simulink model "TST_EngBrk_ECRCtl"  (R2016b)
settings: Solver=FixedStepDiscrete  StartTime=0.0  StopTime=simTime  FixedStep=sampleTime  RelTol=1e-3
values from neighbouring files (symbols this model uses):
  testCase = 1    [initTST_EngBrk_ECRCtl_001.m]    (also in initTST_EngBrk_ECRCtl_002.m = 2; initTST_EngBrk_ECRCtl_003.m = 3; initTST_EngBrk_ECRCtl_004.m = 4)
libraries: simulink x5
settings Model: Creator=WF305  LastModifiedBy=WF305
settings DebuggingCC: SignalRangeChecking=error

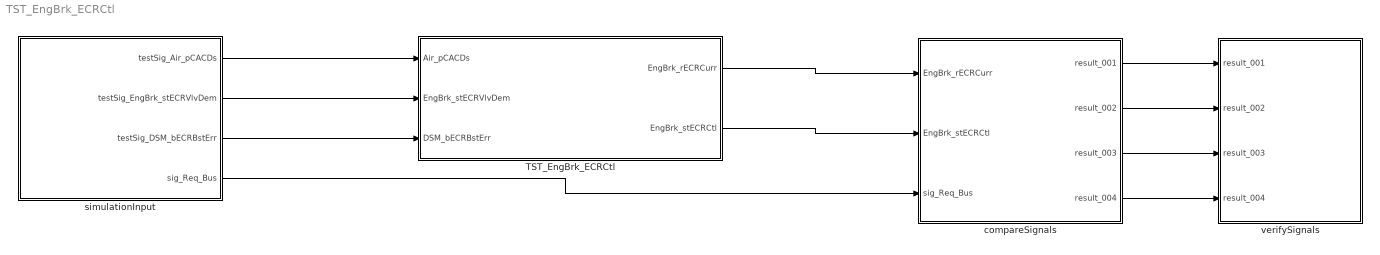
== system TST_EngBrk_ECRCtl ==
  TST_EngBrk_ECRCtl : Subsystem
  compareSignals : Subsystem
  simulationInput : Subsystem
  verifySignals : Subsystem
  wires:
  simulationInput/1(testSig_Air_pCACDs) -> TST_EngBrk_ECRCtl/1(Air_pCACDs)
  simulationInput/2(testSig_EngBrk_stECRVlvDem) -> TST_EngBrk_ECRCtl/2(EngBrk_stECRVlvDem)
  simulationInput/3(testSig_DSM_bECRBstErr) -> TST_EngBrk_ECRCtl/3(DSM_bECRBstErr)
  TST_EngBrk_ECRCtl/1(EngBrk_rECRCurr) -> compareSignals/1(EngBrk_rECRCurr)
  TST_EngBrk_ECRCtl/2(EngBrk_stECRCtl) -> compareSignals/2(EngBrk_stECRCtl)
  simulationInput/4(sig_Req_Bus) -> compareSignals/3(sig_Req_Bus)
  compareSignals/1(result_001) -> verifySignals/1(result_001)
  compareSignals/2(result_002) -> verifySignals/2(result_002)
  compareSignals/3(result_003) -> verifySignals/3(result_003)
  compareSignals/4(result_004) -> verifySignals/4(result_004)

== system TST_EngBrk_ECRCtl/TST_EngBrk_ECRCtl ==
  Air_pCACDs : Inport
  EngBrk_stECRVlvDem : Inport  Port=2
  DSM_bECRBstErr : Inport  Port=3
  EngBrk_ECRCtl : ModelReference  ModelNameDialog=EngBrk_ECRCtl  ModelReferenceVersion=1.8  TriggerPortName=function  TriggerPortTriggerType=function-call  TriggerPortStatesWhenEnabling=held
  Function_Call : simulink/Ports & Subsystems/Function-Call Generator  sample_time=sampleTime  numberOfIterations=1
  EngBrk_rECRCurr : Outport
  EngBrk_stECRCtl : Outport  Port=2
  wires:
  Function_Call/1 -> EngBrk_ECRCtl/Trigger
  Air_pCACDs/1 -> EngBrk_ECRCtl/1
  EngBrk_stECRVlvDem/1 -> EngBrk_ECRCtl/2
  DSM_bECRBstErr/1 -> EngBrk_ECRCtl/3
  EngBrk_ECRCtl/1 -> EngBrk_rECRCurr/1
  EngBrk_ECRCtl/2 -> EngBrk_stECRCtl/1

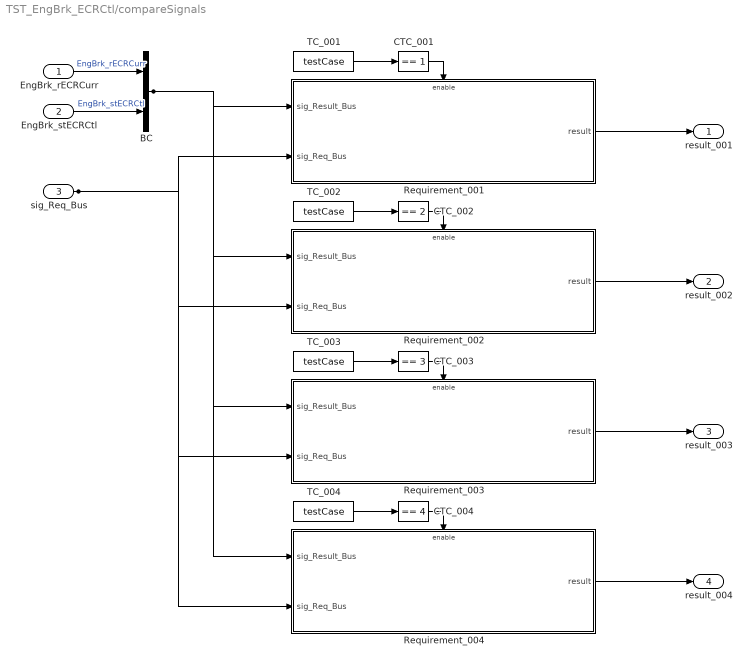
== system TST_EngBrk_ECRCtl/compareSignals ==
  EngBrk_rECRCurr : Inport
  EngBrk_stECRCtl : Inport  Port=2
  sig_Req_Bus : Inport  Port=3
  BC : BusCreator  Inputs=2
  CTC_001 : simulink/Logic and Bit Operations/Compare To Constant  relop===  const=1  OutDataTypeStr=boolean
  CTC_002 : simulink/Logic and Bit Operations/Compare To Constant  relop===  const=2  OutDataTypeStr=boolean
  CTC_003 : simulink/Logic and Bit Operations/Compare To Constant  relop===  const=3  OutDataTypeStr=boolean
  CTC_004 : simulink/Logic and Bit Operations/Compare To Constant  relop===  const=4  OutDataTypeStr=boolean
  Requirement_001 : Subsystem
  Requirement_002 : Subsystem
  Requirement_003 : Subsystem
  Requirement_004 : Subsystem
  TC_001 : Constant  Value=testCase
  TC_002 : Constant  Value=testCase
  TC_003 : Constant  Value=testCase
  TC_004 : Constant  Value=testCase
  result_001 : Outport
  result_002 : Outport  Port=2
  result_003 : Outport  Port=3
  result_004 : Outport  Port=4
  wires:
  EngBrk_rECRCurr/1 -> BC/1  "EngBrk_rECRCurr"
  EngBrk_stECRCtl/1 -> BC/2  "EngBrk_stECRCtl"
  TC_001/1 -> CTC_001/1
  CTC_001/1 -> Requirement_001/Enable
  sig_Req_Bus/1 -> Requirement_001/2(sig_Req_Bus), Requirement_002/2(sig_Req_Bus), Requirement_003/2(sig_Req_Bus), Requirement_004/2(sig_Req_Bus)
  BC/1 -> Requirement_001/1(sig_Result_Bus), Requirement_002/1(sig_Result_Bus), Requirement_003/1(sig_Result_Bus), Requirement_004/1(sig_Result_Bus)
  Requirement_001/1(result) -> result_001/1
  TC_002/1 -> CTC_002/1
  CTC_002/1 -> Requirement_002/Enable
  Requirement_002/1(result) -> result_002/1
  TC_003/1 -> CTC_003/1
  CTC_003/1 -> Requirement_003/Enable
  Requirement_003/1(result) -> result_003/1
  TC_004/1 -> CTC_004/1
  CTC_004/1 -> Requirement_004/Enable
  Requirement_004/1(result) -> result_004/1

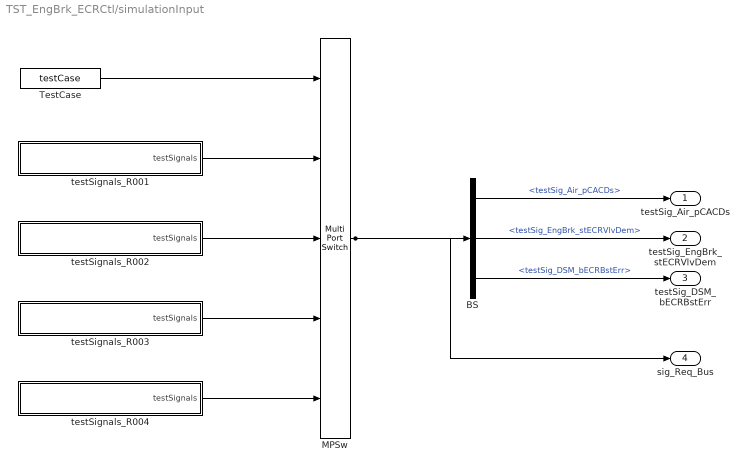
== system TST_EngBrk_ECRCtl/simulationInput ==
  BS : BusSelector  OutputSignals=testSig_Air_pCACDs,testSig_EngBrk_stECRVlvDem,testSig_DSM_bECRBstErr
  MPSw : MultiPortSwitch  Inputs=4  SaturateOnIntegerOverflow=on  InputSameDT=on
  TestCase : Constant  Value=testCase
  testSignals_R001 : Subsystem
  testSignals_R002 : Subsystem
  testSignals_R003 : Subsystem
  testSignals_R004 : Subsystem
  testSig_Air_pCACDs : Outport
  testSig_EngBrk_stECRVlvDem : Outport  Port=2
  testSig_DSM_bECRBstErr : Outport  Port=3
  sig_Req_Bus : Outport  Port=4
  wires:
  BS/1 -> testSig_Air_pCACDs/1  "<testSig_Air_pCACDs>"
  BS/2 -> testSig_EngBrk_stECRVlvDem/1  "<testSig_EngBrk_stECRVlvDem>"
  BS/3 -> testSig_DSM_bECRBstErr/1  "<testSig_DSM_bECRBstErr>"
  MPSw/1 -> BS/1, sig_Req_Bus/1
  TestCase/1 -> MPSw/1
  testSignals_R001/1(testSignals) -> MPSw/2
  testSignals_R002/1(testSignals) -> MPSw/3
  testSignals_R003/1(testSignals) -> MPSw/4
  testSignals_R004/1(testSignals) -> MPSw/5

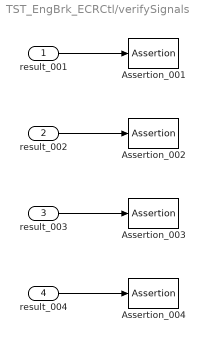
== system TST_EngBrk_ECRCtl/verifySignals ==
  result_001 : Inport
  result_002 : Inport  Port=2
  result_003 : Inport  Port=3
  result_004 : Inport  Port=4
  Assertion_001 : Assertion  Enabled=off
  Assertion_002 : Assertion  Enabled=off
  Assertion_003 : Assertion  Enabled=off
  Assertion_004 : Assertion  Enabled=off
  wires:
  result_001/1 -> Assertion_001/1
  result_002/1 -> Assertion_002/1
  result_003/1 -> Assertion_003/1
  result_004/1 -> Assertion_004/1

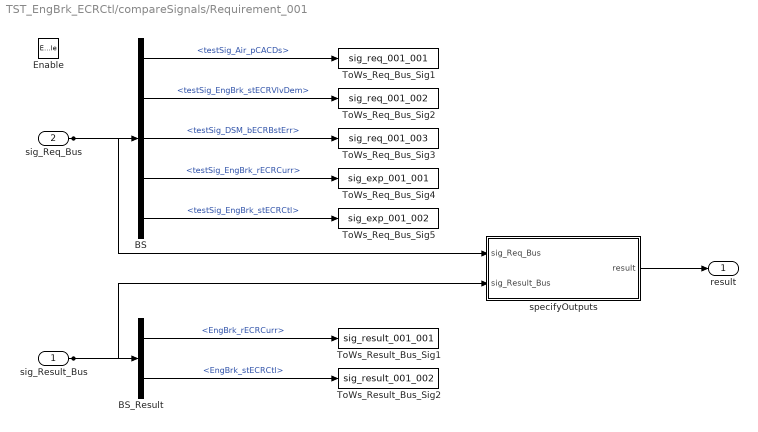
== system TST_EngBrk_ECRCtl/compareSignals/Requirement_001 ==
  sig_Result_Bus : Inport
  sig_Req_Bus : Inport  Port=2
  Enable : EnablePort
  BS : BusSelector  OutputSignals=testSig_Air_pCACDs,testSig_EngBrk_stECRVlvDem,testSig_DSM_bECRBstErr,testSig_EngBrk_rECRCurr,testSig_EngBrk_stECRCtl
  BS_Result : BusSelector  OutputSignals=EngBrk_rECRCurr,EngBrk_stECRCtl
  ToWs_Req_Bus_Sig1 : ToWorkspace  VariableName=sig_req_001_001  SaveFormat=Structure With Time
  ToWs_Req_Bus_Sig2 : ToWorkspace  VariableName=sig_req_001_002  SaveFormat=Structure With Time
  ToWs_Req_Bus_Sig3 : ToWorkspace  VariableName=sig_req_001_003  SaveFormat=Structure With Time
  ToWs_Req_Bus_Sig4 : ToWorkspace  VariableName=sig_exp_001_001  SaveFormat=Structure With Time
  ToWs_Req_Bus_Sig5 : ToWorkspace  VariableName=sig_exp_001_002  SaveFormat=Structure With Time
  ToWs_Result_Bus_Sig1 : ToWorkspace  VariableName=sig_result_001_001  SaveFormat=Structure With Time
  ToWs_Result_Bus_Sig2 : ToWorkspace  VariableName=sig_result_001_002  SaveFormat=Structure With Time
  specifyOutputs : Subsystem
  result : Outport
  wires:
  sig_Req_Bus/1 -> BS/1, specifyOutputs/1(sig_Req_Bus)
  BS/1 -> ToWs_Req_Bus_Sig1/1  "<testSig_Air_pCACDs>"
  BS/2 -> ToWs_Req_Bus_Sig2/1  "<testSig_EngBrk_stECRVlvDem>"
  BS/3 -> ToWs_Req_Bus_Sig3/1  "<testSig_DSM_bECRBstErr>"
  BS/4 -> ToWs_Req_Bus_Sig4/1  "<testSig_EngBrk_rECRCurr>"
  BS/5 -> ToWs_Req_Bus_Sig5/1  "<testSig_EngBrk_stECRCtl>"
  sig_Result_Bus/1 -> BS_Result/1, specifyOutputs/2(sig_Result_Bus)
  BS_Result/1 -> ToWs_Result_Bus_Sig1/1  "<EngBrk_rECRCurr>"
  BS_Result/2 -> ToWs_Result_Bus_Sig2/1  "<EngBrk_stECRCtl>"
  specifyOutputs/1(result) -> result/1

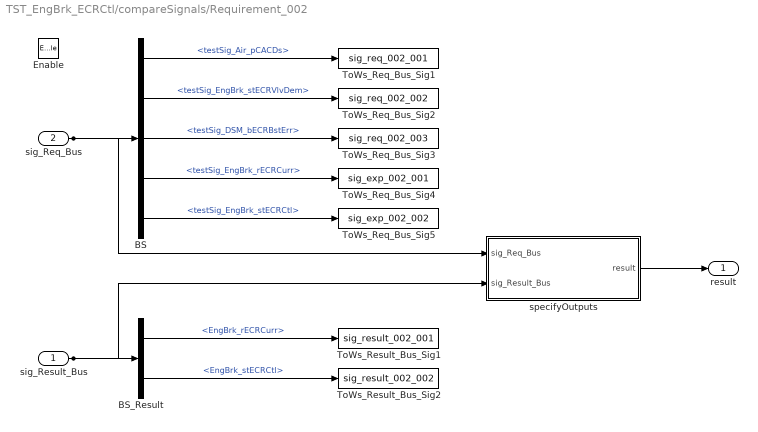
== system TST_EngBrk_ECRCtl/compareSignals/Requirement_002 ==
  sig_Result_Bus : Inport
  sig_Req_Bus : Inport  Port=2
  Enable : EnablePort
  BS : BusSelector  OutputSignals=testSig_Air_pCACDs,testSig_EngBrk_stECRVlvDem,testSig_DSM_bECRBstErr,testSig_EngBrk_rECRCurr,testSig_EngBrk_stECRCtl
  BS_Result : BusSelector  OutputSignals=EngBrk_rECRCurr,EngBrk_stECRCtl
  ToWs_Req_Bus_Sig1 : ToWorkspace  VariableName=sig_req_002_001  SaveFormat=Structure With Time
  ToWs_Req_Bus_Sig2 : ToWorkspace  VariableName=sig_req_002_002  SaveFormat=Structure With Time
  ToWs_Req_Bus_Sig3 : ToWorkspace  VariableName=sig_req_002_003  SaveFormat=Structure With Time
  ToWs_Req_Bus_Sig4 : ToWorkspace  VariableName=sig_exp_002_001  SaveFormat=Structure With Time
  ToWs_Req_Bus_Sig5 : ToWorkspace  VariableName=sig_exp_002_002  SaveFormat=Structure With Time
  ToWs_Result_Bus_Sig1 : ToWorkspace  VariableName=sig_result_002_001  SaveFormat=Structure With Time
  ToWs_Result_Bus_Sig2 : ToWorkspace  VariableName=sig_result_002_002  SaveFormat=Structure With Time
  specifyOutputs : Subsystem
  result : Outport
  wires:
  sig_Req_Bus/1 -> BS/1, specifyOutputs/1(sig_Req_Bus)
  BS/1 -> ToWs_Req_Bus_Sig1/1  "<testSig_Air_pCACDs>"
  BS/2 -> ToWs_Req_Bus_Sig2/1  "<testSig_EngBrk_stECRVlvDem>"
  BS/3 -> ToWs_Req_Bus_Sig3/1  "<testSig_DSM_bECRBstErr>"
  BS/4 -> ToWs_Req_Bus_Sig4/1  "<testSig_EngBrk_rECRCurr>"
  BS/5 -> ToWs_Req_Bus_Sig5/1  "<testSig_EngBrk_stECRCtl>"
  sig_Result_Bus/1 -> BS_Result/1, specifyOutputs/2(sig_Result_Bus)
  BS_Result/1 -> ToWs_Result_Bus_Sig1/1  "<EngBrk_rECRCurr>"
  BS_Result/2 -> ToWs_Result_Bus_Sig2/1  "<EngBrk_stECRCtl>"
  specifyOutputs/1(result) -> result/1

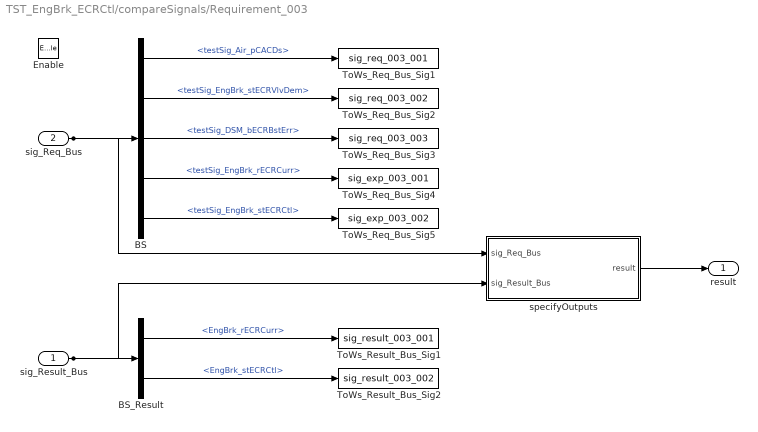
== system TST_EngBrk_ECRCtl/compareSignals/Requirement_003 ==
  sig_Result_Bus : Inport
  sig_Req_Bus : Inport  Port=2
  Enable : EnablePort
  BS : BusSelector  OutputSignals=testSig_Air_pCACDs,testSig_EngBrk_stECRVlvDem,testSig_DSM_bECRBstErr,testSig_EngBrk_rECRCurr,testSig_EngBrk_stECRCtl
  BS_Result : BusSelector  OutputSignals=EngBrk_rECRCurr,EngBrk_stECRCtl
  ToWs_Req_Bus_Sig1 : ToWorkspace  VariableName=sig_req_003_001  SaveFormat=Structure With Time
  ToWs_Req_Bus_Sig2 : ToWorkspace  VariableName=sig_req_003_002  SaveFormat=Structure With Time
  ToWs_Req_Bus_Sig3 : ToWorkspace  VariableName=sig_req_003_003  SaveFormat=Structure With Time
  ToWs_Req_Bus_Sig4 : ToWorkspace  VariableName=sig_exp_003_001  SaveFormat=Structure With Time
  ToWs_Req_Bus_Sig5 : ToWorkspace  VariableName=sig_exp_003_002  SaveFormat=Structure With Time
  ToWs_Result_Bus_Sig1 : ToWorkspace  VariableName=sig_result_003_001  SaveFormat=Structure With Time
  ToWs_Result_Bus_Sig2 : ToWorkspace  VariableName=sig_result_003_002  SaveFormat=Structure With Time
  specifyOutputs : Subsystem
  result : Outport
  wires:
  sig_Req_Bus/1 -> BS/1, specifyOutputs/1(sig_Req_Bus)
  BS/1 -> ToWs_Req_Bus_Sig1/1  "<testSig_Air_pCACDs>"
  BS/2 -> ToWs_Req_Bus_Sig2/1  "<testSig_EngBrk_stECRVlvDem>"
  BS/3 -> ToWs_Req_Bus_Sig3/1  "<testSig_DSM_bECRBstErr>"
  BS/4 -> ToWs_Req_Bus_Sig4/1  "<testSig_EngBrk_rECRCurr>"
  BS/5 -> ToWs_Req_Bus_Sig5/1  "<testSig_EngBrk_stECRCtl>"
  sig_Result_Bus/1 -> BS_Result/1, specifyOutputs/2(sig_Result_Bus)
  BS_Result/1 -> ToWs_Result_Bus_Sig1/1  "<EngBrk_rECRCurr>"
  BS_Result/2 -> ToWs_Result_Bus_Sig2/1  "<EngBrk_stECRCtl>"
  specifyOutputs/1(result) -> result/1

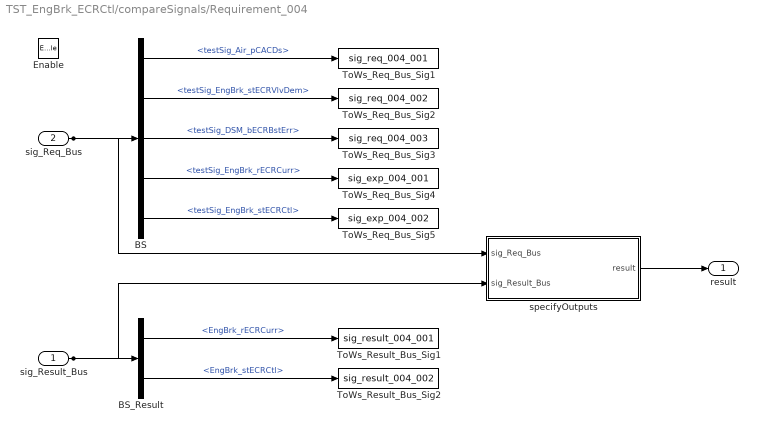
== system TST_EngBrk_ECRCtl/compareSignals/Requirement_004 ==
  sig_Result_Bus : Inport
  sig_Req_Bus : Inport  Port=2
  Enable : EnablePort
  BS : BusSelector  OutputSignals=testSig_Air_pCACDs,testSig_EngBrk_stECRVlvDem,testSig_DSM_bECRBstErr,testSig_EngBrk_rECRCurr,testSig_EngBrk_stECRCtl
  BS_Result : BusSelector  OutputSignals=EngBrk_rECRCurr,EngBrk_stECRCtl
  ToWs_Req_Bus_Sig1 : ToWorkspace  VariableName=sig_req_004_001  SaveFormat=Structure With Time
  ToWs_Req_Bus_Sig2 : ToWorkspace  VariableName=sig_req_004_002  SaveFormat=Structure With Time
  ToWs_Req_Bus_Sig3 : ToWorkspace  VariableName=sig_req_004_003  SaveFormat=Structure With Time
  ToWs_Req_Bus_Sig4 : ToWorkspace  VariableName=sig_exp_004_001  SaveFormat=Structure With Time
  ToWs_Req_Bus_Sig5 : ToWorkspace  VariableName=sig_exp_004_002  SaveFormat=Structure With Time
  ToWs_Result_Bus_Sig1 : ToWorkspace  VariableName=sig_result_004_001  SaveFormat=Structure With Time
  ToWs_Result_Bus_Sig2 : ToWorkspace  VariableName=sig_result_004_002  SaveFormat=Structure With Time
  specifyOutputs : Subsystem
  result : Outport
  wires:
  sig_Req_Bus/1 -> BS/1, specifyOutputs/1(sig_Req_Bus)
  BS/1 -> ToWs_Req_Bus_Sig1/1  "<testSig_Air_pCACDs>"
  BS/2 -> ToWs_Req_Bus_Sig2/1  "<testSig_EngBrk_stECRVlvDem>"
  BS/3 -> ToWs_Req_Bus_Sig3/1  "<testSig_DSM_bECRBstErr>"
  BS/4 -> ToWs_Req_Bus_Sig4/1  "<testSig_EngBrk_rECRCurr>"
  BS/5 -> ToWs_Req_Bus_Sig5/1  "<testSig_EngBrk_stECRCtl>"
  sig_Result_Bus/1 -> BS_Result/1, specifyOutputs/2(sig_Result_Bus)
  BS_Result/1 -> ToWs_Result_Bus_Sig1/1  "<EngBrk_rECRCurr>"
  BS_Result/2 -> ToWs_Result_Bus_Sig2/1  "<EngBrk_stECRCtl>"
  specifyOutputs/1(result) -> result/1

== system TST_EngBrk_ECRCtl/simulationInput/testSignals_R001 ==
  BC : BusCreator  Inputs=5
  spec_Air_pCACDs : FromWorkspace  VariableName=testSig_Air_pCACDs  Interpolate=off  OutputAfterFinalValue=Holding final value
  spec_DSM_bECRBstErr : FromWorkspace  VariableName=testSig_DSM_bECRBstErr  Interpolate=off  OutputAfterFinalValue=Holding final value
  spec_EngBrk_rECRCurr : FromWorkspace  VariableName=testSig_EngBrk_rECRCurr  Interpolate=off  OutputAfterFinalValue=Holding final value
  spec_EngBrk_stECRCtl : FromWorkspace  VariableName=testSig_EngBrk_stECRCtl  Interpolate=off  OutputAfterFinalValue=Holding final value
  spec_EngBrk_stECRVlvDem : FromWorkspace  VariableName=testSig_EngBrk_stECRVlvDem  Interpolate=off  OutputAfterFinalValue=Holding final value
  testSignals : Outport
  wires:
  BC/1 -> testSignals/1
  spec_Air_pCACDs/1 -> BC/1  "testSig_Air_pCACDs"
  spec_EngBrk_stECRVlvDem/1 -> BC/2  "testSig_EngBrk_stECRVlvDem"
  spec_DSM_bECRBstErr/1 -> BC/3  "testSig_DSM_bECRBstErr"
  spec_EngBrk_rECRCurr/1 -> BC/4  "testSig_EngBrk_rECRCurr"
  spec_EngBrk_stECRCtl/1 -> BC/5  "testSig_EngBrk_stECRCtl"

== system TST_EngBrk_ECRCtl/simulationInput/testSignals_R002 ==
  BC : BusCreator  Inputs=5
  spec_Air_pCACDs : FromWorkspace  VariableName=testSig_Air_pCACDs  Interpolate=off  OutputAfterFinalValue=Holding final value
  spec_DSM_bECRBstErr : FromWorkspace  VariableName=testSig_DSM_bECRBstErr  Interpolate=off  OutputAfterFinalValue=Holding final value
  spec_EngBrk_rECRCurr : FromWorkspace  VariableName=testSig_EngBrk_rECRCurr  Interpolate=off  OutputAfterFinalValue=Holding final value
  spec_EngBrk_stECRCtl : FromWorkspace  VariableName=testSig_EngBrk_stECRCtl  Interpolate=off  OutputAfterFinalValue=Holding final value
  spec_EngBrk_stECRVlvDem : FromWorkspace  VariableName=testSig_EngBrk_stECRVlvDem  Interpolate=off  OutputAfterFinalValue=Holding final value
  testSignals : Outport
  wires:
  BC/1 -> testSignals/1
  spec_Air_pCACDs/1 -> BC/1  "testSig_Air_pCACDs"
  spec_EngBrk_stECRVlvDem/1 -> BC/2  "testSig_EngBrk_stECRVlvDem"
  spec_DSM_bECRBstErr/1 -> BC/3  "testSig_DSM_bECRBstErr"
  spec_EngBrk_rECRCurr/1 -> BC/4  "testSig_EngBrk_rECRCurr"
  spec_EngBrk_stECRCtl/1 -> BC/5  "testSig_EngBrk_stECRCtl"

== system TST_EngBrk_ECRCtl/simulationInput/testSignals_R003 ==
  BC : BusCreator  Inputs=5
  spec_Air_pCACDs : FromWorkspace  VariableName=testSig_Air_pCACDs  Interpolate=off  OutputAfterFinalValue=Holding final value
  spec_DSM_bECRBstErr : FromWorkspace  VariableName=testSig_DSM_bECRBstErr  Interpolate=off  OutputAfterFinalValue=Holding final value
  spec_EngBrk_rECRCurr : FromWorkspace  VariableName=testSig_EngBrk_rECRCurr  Interpolate=off  OutputAfterFinalValue=Holding final value
  spec_EngBrk_stECRCtl : FromWorkspace  VariableName=testSig_EngBrk_stECRCtl  Interpolate=off  OutputAfterFinalValue=Holding final value
  spec_EngBrk_stECRVlvDem : FromWorkspace  VariableName=testSig_EngBrk_stECRVlvDem  Interpolate=off  OutputAfterFinalValue=Holding final value
  testSignals : Outport
  wires:
  BC/1 -> testSignals/1
  spec_Air_pCACDs/1 -> BC/1  "testSig_Air_pCACDs"
  spec_EngBrk_stECRVlvDem/1 -> BC/2  "testSig_EngBrk_stECRVlvDem"
  spec_DSM_bECRBstErr/1 -> BC/3  "testSig_DSM_bECRBstErr"
  spec_EngBrk_rECRCurr/1 -> BC/4  "testSig_EngBrk_rECRCurr"
  spec_EngBrk_stECRCtl/1 -> BC/5  "testSig_EngBrk_stECRCtl"

== system TST_EngBrk_ECRCtl/simulationInput/testSignals_R004 ==
  BC : BusCreator  Inputs=5
  spec_Air_pCACDs : FromWorkspace  VariableName=testSig_Air_pCACDs  Interpolate=off  OutputAfterFinalValue=Holding final value
  spec_DSM_bECRBstErr : FromWorkspace  VariableName=testSig_DSM_bECRBstErr  Interpolate=off  OutputAfterFinalValue=Holding final value
  spec_EngBrk_rECRCurr : FromWorkspace  VariableName=testSig_EngBrk_rECRCurr  Interpolate=off  OutputAfterFinalValue=Holding final value
  spec_EngBrk_stECRCtl : FromWorkspace  VariableName=testSig_EngBrk_stECRCtl  Interpolate=off  OutputAfterFinalValue=Holding final value
  spec_EngBrk_stECRVlvDem : FromWorkspace  VariableName=testSig_EngBrk_stECRVlvDem  Interpolate=off  OutputAfterFinalValue=Holding final value
  testSignals : Outport
  wires:
  BC/1 -> testSignals/1
  spec_Air_pCACDs/1 -> BC/1  "testSig_Air_pCACDs"
  spec_EngBrk_stECRVlvDem/1 -> BC/2  "testSig_EngBrk_stECRVlvDem"
  spec_DSM_bECRBstErr/1 -> BC/3  "testSig_DSM_bECRBstErr"
  spec_EngBrk_rECRCurr/1 -> BC/4  "testSig_EngBrk_rECRCurr"
  spec_EngBrk_stECRCtl/1 -> BC/5  "testSig_EngBrk_stECRCtl"

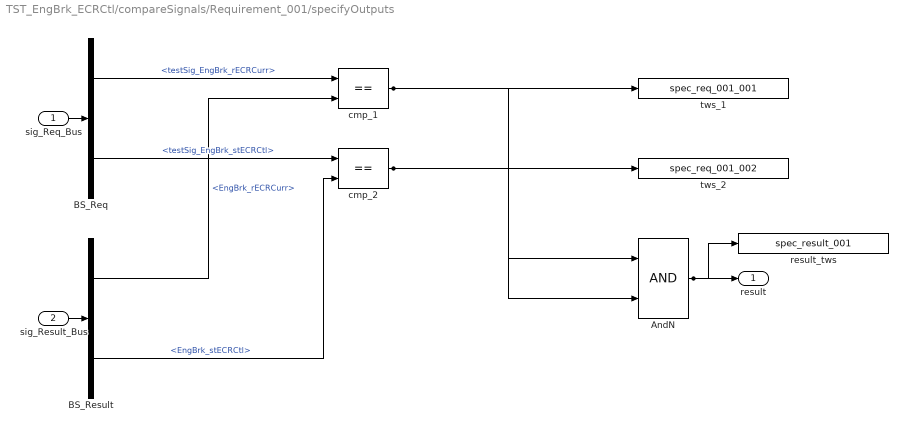
== system TST_EngBrk_ECRCtl/compareSignals/Requirement_001/specifyOutputs ==
  sig_Req_Bus : Inport
  sig_Result_Bus : Inport  Port=2
  AndN : Logic
  BS_Req : BusSelector  OutputSignals=testSig_EngBrk_rECRCurr,testSig_EngBrk_stECRCtl
  BS_Result : BusSelector  OutputSignals=EngBrk_rECRCurr,EngBrk_stECRCtl
  cmp_1 : RelationalOperator  Operator===  RndMeth=Nearest  InputSameDT=on
  cmp_2 : RelationalOperator  Operator===  RndMeth=Nearest  InputSameDT=on
  result_tws : ToWorkspace  VariableName=spec_result_001
  tws_1 : ToWorkspace  VariableName=spec_req_001_001
  tws_2 : ToWorkspace  VariableName=spec_req_001_002
  result : Outport
  wires:
  sig_Req_Bus/1 -> BS_Req/1
  sig_Result_Bus/1 -> BS_Result/1
  AndN/1 -> result/1, result_tws/1
  BS_Req/1 -> cmp_1/1  "<testSig_EngBrk_rECRCurr>"
  BS_Result/1 -> cmp_1/2  "<EngBrk_rECRCurr>"
  cmp_1/1 -> tws_1/1, AndN/1
  BS_Req/2 -> cmp_2/1  "<testSig_EngBrk_stECRCtl>"
  BS_Result/2 -> cmp_2/2  "<EngBrk_stECRCtl>"
  cmp_2/1 -> tws_2/1, AndN/2

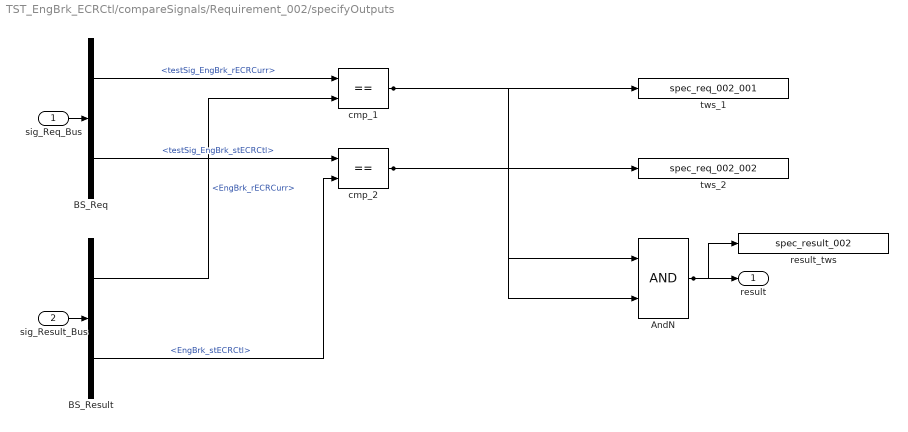
== system TST_EngBrk_ECRCtl/compareSignals/Requirement_002/specifyOutputs ==
  sig_Req_Bus : Inport
  sig_Result_Bus : Inport  Port=2
  AndN : Logic
  BS_Req : BusSelector  OutputSignals=testSig_EngBrk_rECRCurr,testSig_EngBrk_stECRCtl
  BS_Result : BusSelector  OutputSignals=EngBrk_rECRCurr,EngBrk_stECRCtl
  cmp_1 : RelationalOperator  Operator===  RndMeth=Nearest  InputSameDT=on
  cmp_2 : RelationalOperator  Operator===  RndMeth=Nearest  InputSameDT=on
  result_tws : ToWorkspace  VariableName=spec_result_002
  tws_1 : ToWorkspace  VariableName=spec_req_002_001
  tws_2 : ToWorkspace  VariableName=spec_req_002_002
  result : Outport
  wires:
  sig_Req_Bus/1 -> BS_Req/1
  sig_Result_Bus/1 -> BS_Result/1
  AndN/1 -> result/1, result_tws/1
  BS_Req/1 -> cmp_1/1  "<testSig_EngBrk_rECRCurr>"
  BS_Result/1 -> cmp_1/2  "<EngBrk_rECRCurr>"
  cmp_1/1 -> tws_1/1, AndN/1
  BS_Req/2 -> cmp_2/1  "<testSig_EngBrk_stECRCtl>"
  BS_Result/2 -> cmp_2/2  "<EngBrk_stECRCtl>"
  cmp_2/1 -> tws_2/1, AndN/2

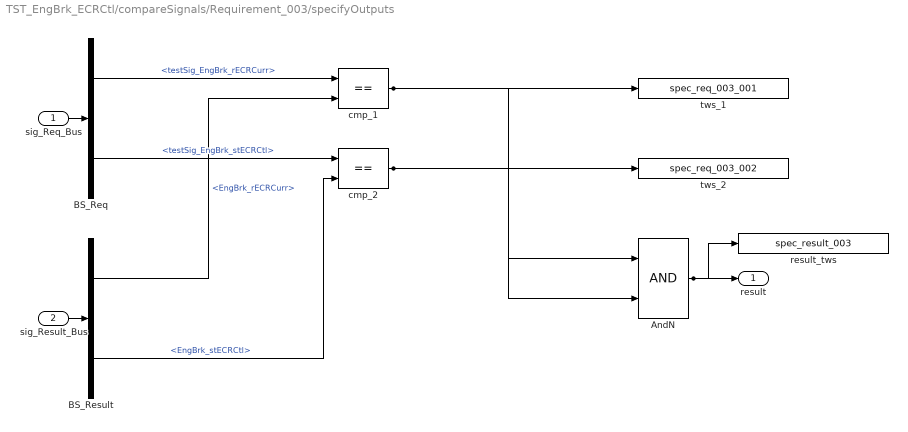
== system TST_EngBrk_ECRCtl/compareSignals/Requirement_003/specifyOutputs ==
  sig_Req_Bus : Inport
  sig_Result_Bus : Inport  Port=2
  AndN : Logic
  BS_Req : BusSelector  OutputSignals=testSig_EngBrk_rECRCurr,testSig_EngBrk_stECRCtl
  BS_Result : BusSelector  OutputSignals=EngBrk_rECRCurr,EngBrk_stECRCtl
  cmp_1 : RelationalOperator  Operator===  RndMeth=Nearest  InputSameDT=on
  cmp_2 : RelationalOperator  Operator===  RndMeth=Nearest  InputSameDT=on
  result_tws : ToWorkspace  VariableName=spec_result_003
  tws_1 : ToWorkspace  VariableName=spec_req_003_001
  tws_2 : ToWorkspace  VariableName=spec_req_003_002
  result : Outport
  wires:
  sig_Req_Bus/1 -> BS_Req/1
  sig_Result_Bus/1 -> BS_Result/1
  AndN/1 -> result/1, result_tws/1
  BS_Req/1 -> cmp_1/1  "<testSig_EngBrk_rECRCurr>"
  BS_Result/1 -> cmp_1/2  "<EngBrk_rECRCurr>"
  cmp_1/1 -> tws_1/1, AndN/1
  BS_Req/2 -> cmp_2/1  "<testSig_EngBrk_stECRCtl>"
  BS_Result/2 -> cmp_2/2  "<EngBrk_stECRCtl>"
  cmp_2/1 -> tws_2/1, AndN/2

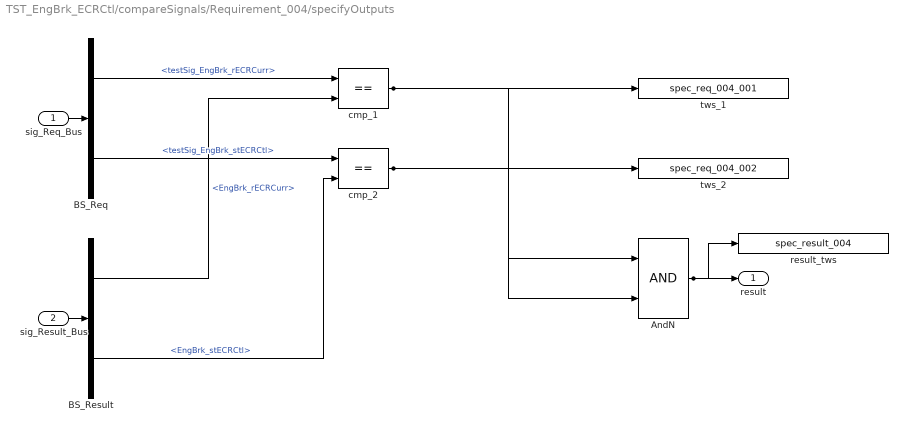
== system TST_EngBrk_ECRCtl/compareSignals/Requirement_004/specifyOutputs ==
  sig_Req_Bus : Inport
  sig_Result_Bus : Inport  Port=2
  AndN : Logic
  BS_Req : BusSelector  OutputSignals=testSig_EngBrk_rECRCurr,testSig_EngBrk_stECRCtl
  BS_Result : BusSelector  OutputSignals=EngBrk_rECRCurr,EngBrk_stECRCtl
  cmp_1 : RelationalOperator  Operator===  RndMeth=Nearest  InputSameDT=on
  cmp_2 : RelationalOperator  Operator===  RndMeth=Nearest  InputSameDT=on
  result_tws : ToWorkspace  VariableName=spec_result_004
  tws_1 : ToWorkspace  VariableName=spec_req_004_001
  tws_2 : ToWorkspace  VariableName=spec_req_004_002
  result : Outport
  wires:
  sig_Req_Bus/1 -> BS_Req/1
  sig_Result_Bus/1 -> BS_Result/1
  AndN/1 -> result/1, result_tws/1
  BS_Req/1 -> cmp_1/1  "<testSig_EngBrk_rECRCurr>"
  BS_Result/1 -> cmp_1/2  "<EngBrk_rECRCurr>"
  cmp_1/1 -> tws_1/1, AndN/1
  BS_Req/2 -> cmp_2/1  "<testSig_EngBrk_stECRCtl>"
  BS_Result/2 -> cmp_2/2  "<EngBrk_stECRCtl>"
  cmp_2/1 -> tws_2/1, AndN/2
